simulink model "auto_tunners"  (R2024b)
settings: Solver=ode23tb  StartTime=0.0  StopTime=200  RelTol=1e-3
undefined symbols (not defined in the file or in its folder): KP_AH, kp_KC, TD_AH, Td_KC, TI_AH, Ti_KC
settings Model: Creator=Esteban Tovar  LastModifiedBy=USUARIO

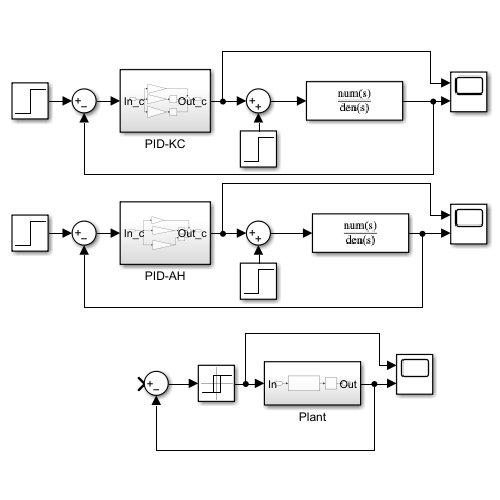
[thumbnail: Simulink's stored preview of the top-level diagram]
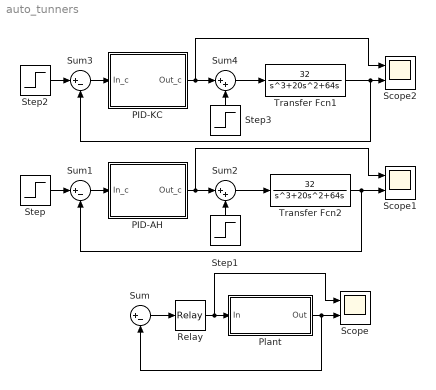
== system auto_tunners ==
  PID-AH : Subsystem
  PID-KC : Subsystem
  Plant : Subsystem
  Relay : Relay  OffOutputValue=-1
  Scope : Scope  NumInputPorts=2
  Scope1 : Scope  NumInputPorts=2
  Scope2 : Scope  NumInputPorts=2
  Step : Step  Time=0  SampleTime=0
  Step1 : Step  Time=100  After=0.5*0.2  SampleTime=0
  Step2 : Step  Time=0  SampleTime=0
  Step3 : Step  Time=100  After=0.5*0.2  SampleTime=0
  Sum : Sum  Inputs=|+-
  Sum1 : Sum  Inputs=|+-
  Sum2 : Sum  Inputs=|++
  Sum3 : Sum  Inputs=|+-
  Sum4 : Sum  Inputs=|++
  Transfer Fcn1 : TransferFcn  Numerator=[32]  Denominator=[1 20 64 0]
  Transfer Fcn2 : TransferFcn  Numerator=[32]  Denominator=[1 20 64 0]
  wires:
  Sum/1 -> Relay/1
  Relay/1 -> Scope/1, Plant/1(In)
  Plant/1(Out) -> Scope/2, Sum/2
  Sum1/1 -> PID-AH/1(In_c)
  Transfer Fcn2/1 -> Scope1/2, Sum1/2
  Step/1 -> Sum1/1
  PID-AH/1(Out_c) -> Sum2/1, Scope1/1
  Sum2/1 -> Transfer Fcn2/1
  Step1/1 -> Sum2/2
  Step2/1 -> Sum3/1
  PID-KC/1(Out_c) -> Sum4/1, Scope2/1
  Transfer Fcn1/1 -> Sum3/2, Scope2/2
  Sum4/1 -> Transfer Fcn1/1
  Sum3/1 -> PID-KC/1(In_c)
  Step3/1 -> Sum4/2

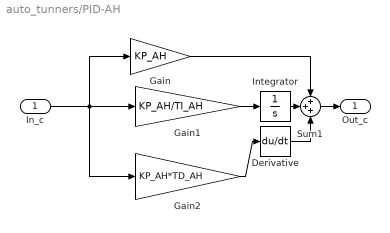
== system auto_tunners/PID-AH ==
  In_c : Inport
  Derivative : Derivative
  Gain : Gain  Gain=KP_AH
  Gain1 : Gain  Gain=KP_AH/TI_AH
  Gain2 : Gain  Gain=KP_AH*TD_AH
  Integrator : Integrator
  Sum1 : Sum  Inputs=+++
  Out_c : Outport
  wires:
  Integrator/1 -> Sum1/2
  In_c/1 -> Gain/1, Gain1/1, Gain2/1
  Gain2/1 -> Derivative/1
  Gain/1 -> Sum1/1
  Gain1/1 -> Integrator/1
  Sum1/1 -> Out_c/1
  Derivative/1 -> Sum1/3

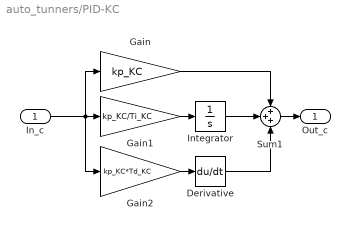
== system auto_tunners/PID-KC ==
  In_c : Inport
  Derivative : Derivative
  Gain : Gain  Gain=kp_KC
  Gain1 : Gain  Gain=kp_KC/Ti_KC
  Gain2 : Gain  Gain=kp_KC*Td_KC
  Integrator : Integrator
  Sum1 : Sum  Inputs=+++
  Out_c : Outport
  wires:
  Integrator/1 -> Sum1/2
  In_c/1 -> Gain2/1, Gain/1, Gain1/1
  Gain2/1 -> Derivative/1
  Gain/1 -> Sum1/1
  Gain1/1 -> Integrator/1
  Sum1/1 -> Out_c/1
  Derivative/1 -> Sum1/3

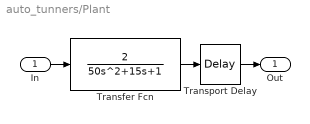
== system auto_tunners/Plant ==
  In : Inport
  Transfer Fcn : TransferFcn  Numerator=[2]  Denominator=[50 15 1]
  Transport Delay : TransportDelay  DelayTime=3
  Out : Outport
  wires:
  In/1 -> Transfer Fcn/1
  Transfer Fcn/1 -> Transport Delay/1
  Transport Delay/1 -> Out/1
